simulink model "AndroidSample"  (R2022a)
settings: Solver=FixedStepAuto  StartTime=0.0  StopTime=10  RelTol=1e-3
values from neighbouring files (symbols this model uses):
  trainedNet_2 = trainNetwork(XTrain,TTrain,layers,options)    [Example.m]
libraries: audiosources x1, deeplib x1
settings Model: Creator=luisb  LastModifiedBy=luisb
settings OptimizationCC: EnhancedBackFolding=on  PassReuseOutputArgsAs=Individual arguments  ZeroExternalMemoryAtStartup=off  ZeroInternalMemoryAtStartup=off  MaxStackSize=64  OptimizeBlockOrder=speed  DifferentSizesBufferReuse=on  OptimizationCustomize=off  EfficientTunableParamExpr=on
settings DebuggingCC: ParameterTunabilityLossMsg=error
settings HardwareCC: ProdBitPerPointer=32  ProdBitPerSizeT=32  ProdBitPerPtrDiffT=32  ProdLargestAtomicInteger=Long  ProdLargestAtomicFloat=Double  ProdWordSize=32  ProdHWDeviceType=ARM Compatible->ARM Cortex  UseEmbeddedCoderFeatures=off
settings SFSimCC: MATLABDynamicMemAlloc=off
settings RTWCC: SystemTargetFile=ert.tlc  HardwareBoard=Android Device  TLCOptions="-aInlineSetEventsForThisBaseRateFcn=TLC_FALSE -aSuppressMultiTaskScheduler=TLC_FALSE  -aRateBasedStepFcn=0"  TemplateMakefile=ert_default_tmf  RTWVerbose=off  Toolchain=Android SDK/NDK Tools
settings CodeAppCC: ForceParamTrailComments=on  IgnoreCustomStorageClasses=off  OperatorAnnotations=on  SimulinkDataObjDesc=on  SFDataObjDesc=on  InsertBlockDesc=on
settings ERTTargetCC: SupportNonInlinedSFcns=on

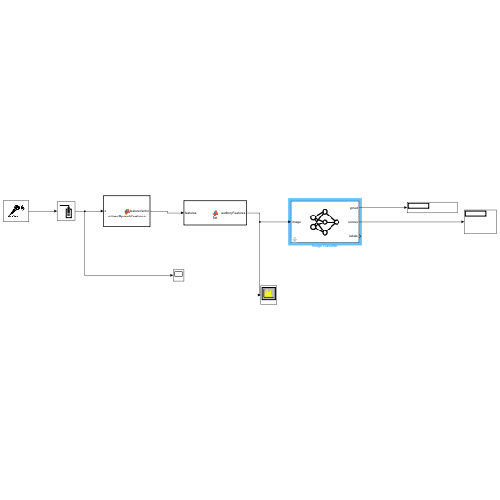
[thumbnail: Simulink's stored preview of the top-level diagram]
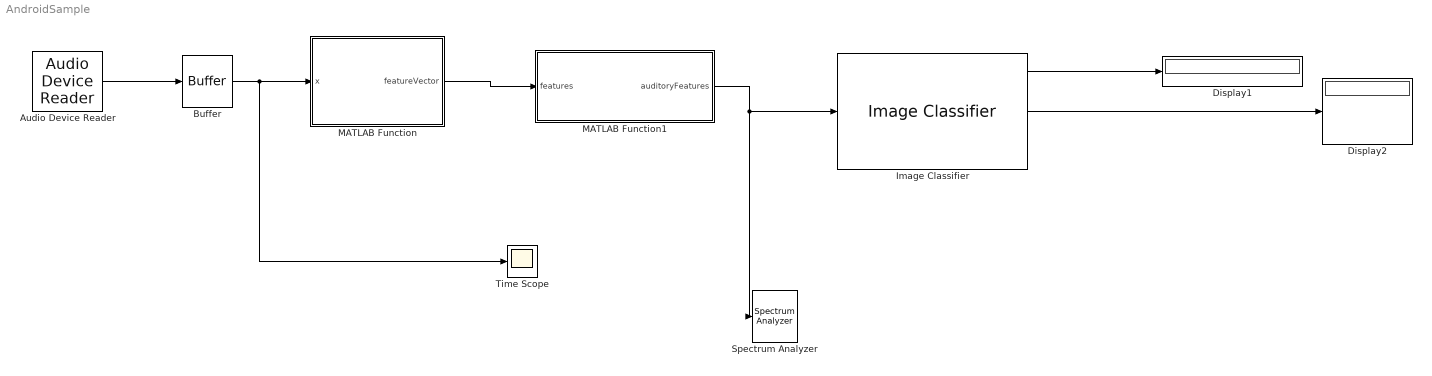
== system AndroidSample ==
  Audio Device Reader : audiosources/Audio Device Reader  Driver=DirectSound  Device=Default  SampleRate=44100  NumChannels=1  SamplesPerFrame=1024  BitDepth=16-bit integer  NumBuffers=10  DefaultInputChannelMapping=on  InputChannelMapping=1:2  OutputNumOverrunSamples=off  OutputDataType=double  DriverIdx=1  DeviceWarnFlag=''
      settings: SourceProductBaseCode=AU
  Buffer : Buffer  N=16000  V=10  OutputFrames=off
  Display1 : Display
  Display2 : Display
  Image Classifier : deeplib/Image Classifier  Network=Network from MAT-file  NetworkFunction=squeezenet  NetworkFilePath=C:\Users\luisb\OneDrive\Documents\Audio_Classification\trainedNet_2.mat  MiniBatchSize=128  ResizeInput=on  Classification=on  Predictions=on  ForceInterpretedSim=off  PredictMode=All probabilities and labels  K=5
      settings: SourceProductBaseCode=NN
  MATLAB Function : MATLAB Function  TreatAsAtomicUnit=on
  MATLAB Function1 : MATLAB Function  TreatAsAtomicUnit=on
  Spectrum Analyzer : SpectrumAnalyzer
  Time Scope : Scope
  wires:
  Audio Device Reader/1 -> Buffer/1
  Buffer/1 -> Time Scope/1, MATLAB Function/1(x)
  MATLAB Function1/1(auditoryFeatures) -> Spectrum Analyzer/1, Image Classifier/1
  MATLAB Function/1(featureVector) -> MATLAB Function1/1(features)
  Image Classifier/1 -> Display1/1
  Image Classifier/2 -> Display2/1

== matlab function AndroidSample/MATLAB Function ==
  data: x input; featureVector output
function featureVector = extractSpeechFeatures(x)
%extractSpeechFeatures Extract multiple features from batch audio
%   featureVector = extractSpeechFeatures(audioIn) returns audio features
%   extracted from audioIn.
%
%   Parameters of the audioFeatureExtractor used to generate this
%   function must be honored when calling this function.
%    - Sample rate of the input should be 16000 Hz.
%    - Input frame length should be greater than or equal to 240 samples.
%
%
%      % EXAMPLE 1: Extract features
%        source = dsp.ColoredNoise("SamplesPerFrame",16000);
%        for ii = 1:10
%            audioIn = source();
%            featureArray = extractSpeechFeatures(audioIn);
%            % ... do something with featureArray ...
%        end
%
%
%      % EXAMPLE 2: Generate code
%        targetDataType = "single";
%        codegen extractSpeechFeatures -args {ones(16000,1,targetDataType)}
%        source = dsp.ColoredNoise("SamplesPerFrame",16000, ...
%                                  "OutputDataType",targetDataType);
%        for ii = 1:10
%            audioIn = source();
%            featureArray = extractSpeechFeatures_mex(audioIn);
%            % ... do something with featureArray ...
%        end
%
%   See also audioFeatureExtractor, dsp.AsyncBuffer, codegen.

%   Generated by audioFeatureExtractor on 21-Feb-2023 09:47:32 -0600
%#codegen

dataType = underlyingType(x);
[numSamples,numChannels] = size(x);

props = coder.const(getProps(dataType));

persistent config outputIndex
if isempty(outputIndex)
    [config, outputIndex] = coder.const(@getConfig,dataType,props);
end

% Preallocate feature vector
numHops = floor((numSamples-numel(props.Window))/(numel(props.Window) - props.OverlapLength)) + 1;
featureVector = coder.nullcopy(zeros(numHops,props.NumFeatures,numChannels,dataType));

% Short-time Fourier transform
Y = stft(x,"Window",props.Window,"OverlapLength",props.OverlapLength,"FFTLength",props.FFTLength,"FrequencyRange","onesided");
Z = reshape(Y,[],numHops*numChannels);
Zpower = real(Z.*conj(Z));

% Bark spectrum
barkSpectrum = reshape(config.barkSpectrum.FilterBank*Zpower,[],numHops,numChannels);
featureVector(:,outputIndex.barkSpectrum,:) = permute(barkSpectrum,[2,1,3]);
end

function props = getProps(dataType)
props.Window = cast([0;0.00017133751222137005854051494679879;0.0007852326227130833835587964131264;0.0015413331334360180768783266103128;0.0027390523158633550693252800556365;0.0042775693130948089226706088084029;0.0061558297024311148248898462043144;0.0083725462180226917219272309012013;0.010926199633097155583527637645602;0.013815039801161721477740229602205;0.017037086855465843893142618981074;0.020590132565903473960133851505816;0.024471741852423234409030783353955;0.028679254453910785205295042032958;0.033209786751399128501560653603519;0.038060233744356630758431947469944;0.043227271178699566700487366688321;0.048707357825069685919316953004454;0.054496737905816050595575461557019;0.060591443669017308604196614396642;0.066987298107780646194697737882962;0.073679917822953855388590227448731;0.080664716027287974853265950514469;0.087936905688992206275855778585537;0.095491502812526274368565282202326;0.10332332985438241745868026555399;0.11142701927151460461473675422894;0.11979701719998453457449727466155;0.12842758726130287794120476974058;0.13731281449385612791758148887311;0.14644660940672621363134453531529;0.15582271215312304413203037256608;0.16543469682057088121496235544328;0.17527597583490822641394402126025;0.18533980447508124900224402153981;0.19561928549563967205671133342548;0.20610737385376343144827160358545;0.21679688153758358559741736826254;0.22768048249248640235720131386188;0.23875071764202554502887210219342;0.24999999999999994448884876874217;0.26142061987019582502966841275338;0.27300475013022657000405502003559;0.28474445159585237696830972708995;0.29663167846209981259875121395453;0.30865828381745508135480804412509;0.32081602522734992133379705592233;0.33309657038311457633028567215661;0.34549150281252627436856528220233;0.3579923276480386218345586257783;0.37059047744873963026179808366578;0.38327731807204723502024990011705;0.3960441545911204119789772448712;0.40888223725392613960849530485575;0.42178276747988452388682389937458;0.43473690388997415778860045065812;0.447735768366173292331922084486;0.46077045213607747964346117441892;0.47383202187852802023115827978472;0.48691152584606334219330392443226;0.49999999999999994448884876874217;0.51308847415393654678439361305209;0.52616797812147186874653925769962;0.53922954786392240933423636306543;0.55226423163382665215692668425618;0.5652630961100256756779458555684;0.57821723252011547611317610062542;0.5911177627460737493692022326286;0.6039558454088795880210227551288;0.61672268192795254293514517485164;0.62940952255126036973820191633422;0.64200767235196132265429014296387;0.65450849718747372563143471779767;0.66690342961688542366971432784339;0.67918397477265013417735417533549;0.69134171618254480762288949335925;0.70336832153790007637894632352982;0.71525554840414762303169027291005;0.72699524986977337448479374870658;0.73857938012980417497033158724662;0.74999999999999988897769753748435;0.76124928235797439945997666654876;0.77231951750751348662049622362247;0.78320311846241630338028016922181;0.79389262614623645752942593389889;0.80438071450436032794328866657452;0.81466019552491863997545351594454;0.82472402416509171807490474748192;0.83456530317942889674043271952542;0.84417728784687706689027208994958;0.85355339059327373085750423342688;0.86268718550614376106011604861123;0.87157241273869723308109769277507;0.88020298280001540991435149408062;0.88857298072848545089641447702888;0.89667667014561747151901727193035;0.90450849718747372563143471779767;0.91206309431100784923529545267229;0.91933528397271202514673404948553;0.92632008217704608910025854129344;0.93301270189221940931645349337487;0.93940855633098263588465215434553;0.94550326209418389389327330718515;0.95129264217493014754722935322206;0.95677272882130048881066386456951;0.96193976625564336924156805253006;0.96679021324860081598728811513865;0.97132074554608927030585618922487;0.97552825814757682110212044790387;0.97940986743409652603986614849418;0.9829629131445341005957061497611;0.9861849601988382785222597703978;0.9890738003669028444164723623544;0.99162745378197725276692153784097;0.99384417029756888517511015379569;0.99572243068690524658848062244942;0.99726094768413664493067471994436;0.99845866686656403743427290464751;0.99931476737728686110528997232905;0.99982866248777857443030825379537;1;0.99982866248777857443030825379537;0.99931476737728686110528997232905;0.99845866686656403743427290464751;0.99726094768413664493067471994436;0.99572243068690524658848062244942;0.99384417029756888517511015379569;0.99162745378197725276692153784097;0.9890738003669028444164723623544;0.9861849601988382785222597703978;0.9829629131445341005957061497611;0.97940986743409652603986614849418;0.97552825814757682110212044790387;0.97132074554608927030585618922487;0.96679021324860081598728811513865;0.96193976625564336924156805253006;0.95677272882130048881066386456951;0.95129264217493014754722935322206;0.94550326209418389389327330718515;0.93940855633098263588465215434553;0.93301270189221940931645349337487;0.92632008217704608910025854129344;0.91933528397271202514673404948553;0.91206309431100784923529545267229;0.90450849718747372563143471779767;0.89667667014561747151901727193035;0.88857298072848545089641447702888;0.88020298280001540991435149408062;0.87157241273869723308109769277507;0.86268718550614376106011604861123;0.85355339059327373085750423342688;0.84417728784687706689027208994958;0.83456530317942889674043271952542;0.82472402416509171807490474748192;0.81466019552491863997545351594454;0.80438071450436032794328866657452;0.79389262614623645752942593389889;0.78320311846241630338028016922181;0.77231951750751348662049622362247;0.76124928235797439945997666654876;0.74999999999999988897769753748435;0.73857938012980417497033158724662;0.72699524986977337448479374870658;0.71525554840414762303169027291005;0.70336832153790007637894632352982;0.69134171618254480762288949335925;0.67918397477265013417735417533549;0.66690342961688542366971432784339;0.65450849718747372563143471779767;0.64200767235196132265429014296387;0.62940952255126036973820191633422;0.61672268192795254293514517485164;0.6039558454088795880210227551288;0.5911177627460737493692022326286;0.57821723252011547611317610062542;0.5652630961100256756779458555684;0.55226423163382665215692668425618;0.53922954786392240933423636306543;0.52616797812147186874653925769962;0.51308847415393654678439361305209;0.49999999999999994448884876874217;0.48691152584606334219330392443226;0.47383202187852802023115827978472;0.46077045213607747964346117441892;0.447735768366173292331922084486;0.43473690388997415778860045065812;0.42178276747988452388682389937458;0.40888223725392613960849530485575;0.3960441545911204119789772448712;0.38327731807204723502024990011705;0.37059047744873963026179808366578;0.3579923276480386218345586257783;0.34549150281252627436856528220233;0.33309657038311457633028567215661;0.32081602522734992133379705592233;0.30865828381745508135480804412509;0.29663167846209981259875121395453;0.28474445159585237696830972708995;0.27300475013022657000405502003559;0.26142061987019582502966841275338;0.24999999999999994448884876874217;0.23875071764202554502887210219342;0.22768048249248640235720131386188;0.21679688153758358559741736826254;0.20610737385376343144827160358545;0.19561928549563967205671133342548;0.18533980447508124900224402153981;0.17527597583490822641394402126025;0.16543469682057088121496235544328;0.15582271215312304413203037256608;0.14644660940672621363134453531529;0.13731281449385612791758148887311;0.12842758726130287794120476974058;0.11979701719998453457449727466155;0.11142701927151460461473675422894;0.10332332985438241745868026555399;0.095491502812526274368565282202326;0.087936905688992206275855778585537;0.080664716027287974853265950514469;0.073679917822953855388590227448731;0.066987298107780646194697737882962;0.060591443669017308604196614396642;0.054496737905816050595575461557019;0.048707357825069685919316953004454;0.043227271178699566700487366688321;0.038060233744356630758431947469944;0.033209786751399128501560653603519;0.028679254453910785205295042032958;0.024471741852423234409030783353955;0.020590132565903473960133851505816;0.017037086855465843893142618981074;0.013815039801161721477740229602205;0.010926199633097155583527637645602;0.0083725462180226917219272309012013;0.0061558297024311148248898462043144;0.0042775693130948089226706088084029;0.0027390523158633550693252800556365;0.0015413331334360180768783266103128;0.0006852326227130833835587964131264;0.00017133751222137005854051494679879],dataType);
props.OverlapLength = cast(124,dataType);
props.SampleRate = cast(16000,dataType);
props.FFTLength = uint16(1024);
props.NumFeatures = uint8(50);
end

function [config, outputIndex] = getConfig(dataType, props)

barkFilterbank = designAuditoryFilterBank(props.SampleRate, ...
    "FrequencyScale","bark", ...
    "FFTLength",props.FFTLength, ...
    "OneSided",true, ...
    "FrequencyRange",[0 8000], ...
    "NumBands",50, ...
    "Normalization","bandwidth", ...
    "FilterBankDesignDomain","linear");
config.barkSpectrum.FilterBank = cast(barkFilterbank,dataType);

outputIndex.barkSpectrum = uint8(1:50);
end

== matlab function AndroidSample/MATLAB Function1 ==
  data: features input; auditoryFeatures output
function auditoryFeatures = fcn(features)
auditoryFeatures = log10(features + 1e-6);
end
